simulink model "detection_and_isolation_v3"  (R2018a)
settings: Solver=ode45  StartTime=0.0  StopTime=0.8  RelTol=1e-3
values from neighbouring files (symbols this model uses):
  Ad = sysd.A    [SimulinkInit.m]
  Bd = sysd.B    [SimulinkInit.m]
  C1 = Cd(1,:)    [SimulinkInit.m]
  C2 = Cd(2,:)    [SimulinkInit.m]
  C3 = Cd(3,:)    [SimulinkInit.m]
  C4 = Cd(4,:)    [SimulinkInit.m]
  Cd = sysd.C    [SimulinkInit.m]
  T1 = 0.4    [parametros_BIO.m]
  T2 = 1    [parametros_BIO.m]
  T3 = 15    [parametros_BIO.m]
  T4 = 2.5    [parametros_BIO.m]
  T5 = 3.3    [parametros_BIO.m]
  tm = 1e-4    (= 0.0001)    [SimulinkInit.m]
undefined symbols (not defined in the file or in its folder): C10, C11, C12, C5, C6, C7, C8, C9, F1, F10, F11, F12, F2, F3, F4, F5, F6, F7, F8, F9, H1, H10, H11, H12, H2, H3, H4, H5, H6, H7, H8, H9, K10U, K11U, K12U, K1U, K2U, K3U, K4U, K5U, K6U, K7U, K8U, K9U, T10, T11, T12, T6, T7, T8, T9
libraries: dsparch4 x2, powerlib_meascontrol x2, dspstat3 x2, dspmlti4 x1
settings Model: Creator=cmparedes  LastModifiedBy=cmparedes

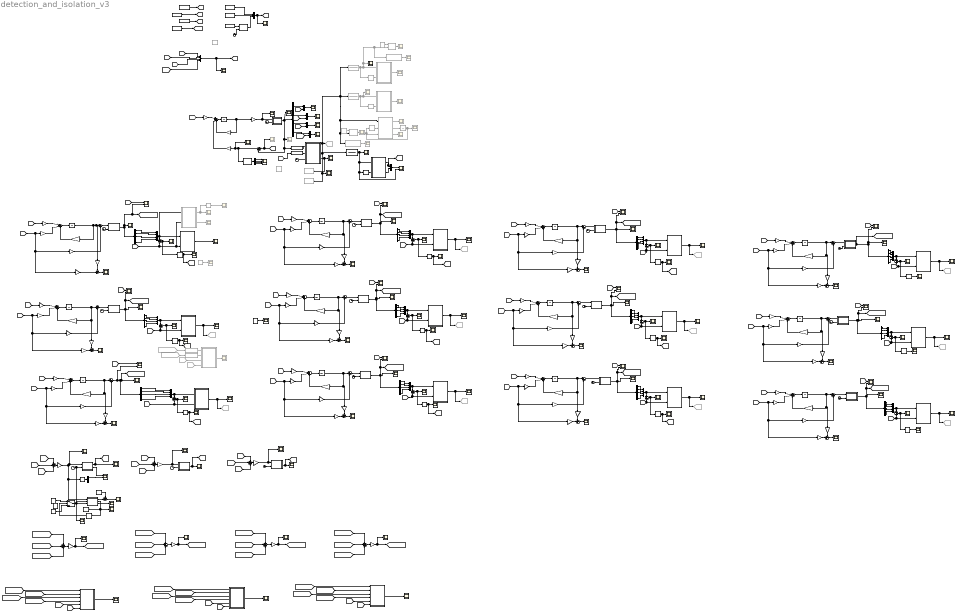
== system detection_and_isolation_v3 ==
  Abs : Abs
  Array From Workspace1 : FromWorkspace  VariableName=[tiempo,I2]  SampleTime=tm
  Array From Workspace2 : FromWorkspace  VariableName=[tiempo,I1]  SampleTime=tm
  Array From Workspace3 : FromWorkspace  VariableName=[tiempo,I3]  SampleTime=tm
  Array From Workspace4 : FromWorkspace  VariableName=[tiempo,V_load]  SampleTime=tm
  Array From Workspace5 : FromWorkspace  VariableName=[tiempo,u1]  SampleTime=tm
  Array From Workspace6 : FromWorkspace  VariableName=[tiempo,u2]  SampleTime=tm
  Array From Workspace7 : FromWorkspace  VariableName=[tiempo,u3]  SampleTime=tm
  Clock{,1..16} (17 alike) : Clock
  Constant : Constant  Value=0
  Constant1 : Constant
  Constant2 : Constant
  Constant3 : Constant
  Constant8 : Constant  Commented=on  Value=10
  Constant9 : Constant  Commented=on  Value=10
  DWT : dspmlti4/Dyadic Analysis Filter Bank  Commented=on  Wname=User-defined  OrdRec_ordDec=[1 / 1]  Order=2  LPF="[0.0352   -0.0854   -0.1350   0.4599   0.8069   0.3327]"  HPF="[-0.3327    0.8069   -0.4599   -0.1350    0.0854    0.0352]"  NumLevels=2  tree=Symmetric  Output=Single port  OutputFrames=off
      settings: SourceProductName=DSP System Toolbox  SourceProductBaseCode=DS
  Delay : Delay  Commented=on  DelayLength=1
  Delay1 : Delay  Commented=on  DelayLength=1
  Delay2 : Delay  DelayLength=1
  Delay3 : Delay  Commented=on  DelayLength=1
  Delay4 : Delay  DelayLength=1
  Demux : Demux
  Demux{1,3..13} (12 alike) : Demux  Outputs=5
  Demux19 : Demux
  Demux2 : Demux
  Derivative{,1..2,4..12} (12 alike) : Derivative  CoefficientInTFapproximation=0
  Derivative13 : Derivative  Commented=on  CoefficientInTFapproximation=0
  Derivative3 : Derivative
  From54 : From  Commented=on  GotoTag=x_hat_uio1
  From55 : From  Commented=on  GotoTag=x_hat_uio2
  From56 : From  Commented=on  GotoTag=rol
  From57 : From  Commented=on  GotoTag=ruo2
  Gain{,1..6} (7 alike) : Gain  Gain=1/3
  Goto{5,7,9,11,13,15,17,19,36} (9 alike) : Goto  Commented=on  GotoTag=ruo4
  Goto28 : Goto  Commented=on  GotoTag=ruo2
  Goto31 : Goto  Commented=on  GotoTag=ruo3
  Goto35 : Goto  Commented=on  GotoTag=rol
  Hw4 : dsparch4/Analog Filter Design  Commented=on  method=Bessel  filttype=Lowpass  N=2  Wlo=7000*2*pi  Whi=80  Rp=2  Rs=80
  Hw5 : dsparch4/Analog Filter Design  Commented=on  method=Bessel  filttype=Lowpass  N=20  Wlo=60*2*pi  Whi=80  Rp=2  Rs=80
  Integrator : Integrator  Commented=on
  MATLAB Function : MATLAB Function  TreatAsAtomicUnit=on
  MATLAB Function1 : MATLAB Function  TreatAsAtomicUnit=on
  MATLAB Function10 : MATLAB Function  TreatAsAtomicUnit=on
  MATLAB Function11 : MATLAB Function  Commented=on  TreatAsAtomicUnit=on
  MATLAB Function12 : MATLAB Function  TreatAsAtomicUnit=on
  MATLAB Function13 : MATLAB Function  TreatAsAtomicUnit=on
  MATLAB Function14 : MATLAB Function  Commented=on  TreatAsAtomicUnit=on
  MATLAB Function15 : MATLAB Function  TreatAsAtomicUnit=on
  MATLAB Function16 : MATLAB Function  TreatAsAtomicUnit=on
  MATLAB Function17 : MATLAB Function  TreatAsAtomicUnit=on
  MATLAB Function18 : MATLAB Function  TreatAsAtomicUnit=on
  MATLAB Function19 : MATLAB Function  TreatAsAtomicUnit=on
  MATLAB Function2 : MATLAB Function  TreatAsAtomicUnit=on
  MATLAB Function20 : MATLAB Function  TreatAsAtomicUnit=on
  MATLAB Function21 : MATLAB Function  TreatAsAtomicUnit=on
  MATLAB Function22 : MATLAB Function  TreatAsAtomicUnit=on
  MATLAB Function23 : MATLAB Function  TreatAsAtomicUnit=on
  MATLAB Function24 : MATLAB Function  TreatAsAtomicUnit=on
  MATLAB Function25 : MATLAB Function  TreatAsAtomicUnit=on
  MATLAB Function26 : MATLAB Function  TreatAsAtomicUnit=on
  MATLAB Function27 : MATLAB Function  TreatAsAtomicUnit=on
  MATLAB Function28 : MATLAB Function  TreatAsAtomicUnit=on
  MATLAB Function29 : MATLAB Function  TreatAsAtomicUnit=on
  MATLAB Function3 : MATLAB Function  TreatAsAtomicUnit=on
  MATLAB Function30 : MATLAB Function  TreatAsAtomicUnit=on
  MATLAB Function31 : MATLAB Function  TreatAsAtomicUnit=on
  MATLAB Function32 : MATLAB Function  TreatAsAtomicUnit=on
  MATLAB Function33 : MATLAB Function  TreatAsAtomicUnit=on
  MATLAB Function34 : MATLAB Function  TreatAsAtomicUnit=on
  MATLAB Function35 : MATLAB Function  TreatAsAtomicUnit=on
  MATLAB Function36 : MATLAB Function  TreatAsAtomicUnit=on
  MATLAB Function37 : MATLAB Function  TreatAsAtomicUnit=on
  MATLAB Function38 : MATLAB Function  TreatAsAtomicUnit=on
  MATLAB Function39 : MATLAB Function  TreatAsAtomicUnit=on
  MATLAB Function4 : MATLAB Function  Commented=on  TreatAsAtomicUnit=on
  MATLAB Function5 : MATLAB Function  Commented=on  TreatAsAtomicUnit=on
  MATLAB Function6 : MATLAB Function  Commented=on  TreatAsAtomicUnit=on
  MATLAB Function7 : MATLAB Function  TreatAsAtomicUnit=on
  MATLAB Function8 : MATLAB Function  TreatAsAtomicUnit=on
  MATLAB Function9 : MATLAB Function  TreatAsAtomicUnit=on
  Mean (Variable Frequency) : powerlib_meascontrol/Measurements/Mean (Variable Frequency)  Commented=on  Finit=60  Fmin=45  Vinit=0  Ts=0
      settings: SourceProductName=Simscape Power Systems  SourceProductBaseCode=PS
  Mean (Variable Frequency)1 : powerlib_meascontrol/Measurements/Mean (Variable Frequency)  Commented=on  Finit=60  Fmin=45  Vinit=0  Ts=0
      settings: SourceProductName=Simscape Power Systems  SourceProductBaseCode=PS
  Median Filter : dspstat3/Median Filter  Commented=on  WindowLength=100  SimulateUsing=Interpreted execution
      settings: SourceProductName=DSP System Toolbox  SourceProductBaseCode=DS
  Median Filter1 : dspstat3/Median Filter  Commented=on  WindowLength=100  SimulateUsing=Interpreted execution
      settings: SourceProductName=DSP System Toolbox  SourceProductBaseCode=DS
  Memory : Memory
  Mux{1..6,8,13,15..19} (13 alike) : Mux
  Mux{9..12,14} (5 alike) : Mux  Inputs=2
  Mux7 : Mux  Inputs=3
  Scope{,1,4..7,9..13,15,23..25,27..32,34..39,41,44..56,58..77,84,93..104,106..122} (91 alike) : Scope
  Scope{2..3,8,14,16..22,26,33,40,57,92,105} (17 alike) : Scope  Commented=on
  Scope{42,78..83,85..91} (14 alike) : Scope  NumInputPorts=2
  Scope43 : Scope  NumInputPorts=4
  Signal Specification : SignalSpecification  Dimensions=4
  Signal Specification1 : SignalSpecification  Dimensions=4
  Signal Specification2 : SignalSpecification  Commented=on  Dimensions=3
  Signal Specification3 : SignalSpecification  Commented=on  Dimensions=3
  Sum{,3,7,15,18,22,30,34,36,42,46,48} (12 alike) : Sum  Inputs=|++
  Sum{1..2,5,11,13,20,26,28,32,38,40,44} (12 alike) : Sum  Inputs=+-
  Sum10 : Sum  Inputs=|+-
  Sum{6,12,17,21,23..24,27,29,33,39,41,45} (12 alike) : Sum  Inputs=-+|
  Sum{4,8..9,14,16,19,25,31,35,37,43,47,49} (13 alike) : Sum  Inputs=|+++  SampleTime=tm
  Sum{50..52,54..57} (7 alike) : Sum  Inputs=+++
  Sum53 : Sum  Inputs=+-|
  Switch : Switch  Criteria=u2 > Threshold
  To Workspace : ToWorkspace  Commented=on  VariableName=det  SampleTime=1e-4
  To Workspace1 : ToWorkspace  Commented=on  VariableName=norm  SampleTime=1e-4
  Transfer Fcn : TransferFcn  Commented=on  Denominator=[0.025 1]
  Transfer Fcn5 : TransferFcn  Commented=on  Denominator=[0.0025 1]
  Transfer Fcn6 : TransferFcn  Denominator=[0.005 1]
  Unit Delay{1..13} (13 alike) : UnitDelay  SampleTime=tm
  adis1 : Gain  Gain=F3  Multiplication=Matrix(K*u) (u vector)  SampleTime=tm
  adis10 : Gain  Gain=Ld'  Multiplication=Matrix(K*u) (u vector)  SampleTime=tm
  adis11 : Gain  Gain=F1  Multiplication=Matrix(K*u) (u vector)  SampleTime=tm
  adis12 : Gain  Gain=F2  Multiplication=Matrix(K*u) (u vector)  SampleTime=tm
  adis13 : Gain  Gain=F11  Multiplication=Matrix(K*u) (u vector)  SampleTime=tm
  adis14 : Gain  Gain=F12  Multiplication=Matrix(K*u) (u vector)  SampleTime=tm
  adis2 : Gain  Gain=F4  Multiplication=Matrix(K*u) (u vector)  SampleTime=tm
  adis3 : Gain  Gain=F5  Multiplication=Matrix(K*u) (u vector)  SampleTime=tm
  adis4 : Gain  Gain=F6  Multiplication=Matrix(K*u) (u vector)  SampleTime=tm
  adis5 : Gain  Gain=F7  Multiplication=Matrix(K*u) (u vector)  SampleTime=tm
  adis6 : Gain  Gain=F8  Multiplication=Matrix(K*u) (u vector)  SampleTime=tm
  adis7 : Gain  Gain=Ad  Multiplication=Matrix(K*u) (u vector)  SampleTime=tm
  adis8 : Gain  Gain=F9  Multiplication=Matrix(K*u) (u vector)  SampleTime=tm
  adis9 : Gain  Gain=F10  Multiplication=Matrix(K*u) (u vector)  SampleTime=tm
  bdis1 : Gain  Gain=T3*Bd  Multiplication=Matrix(K*u) (u vector)  SampleTime=tm
  bdis10 : Gain  Gain=T2*Bd  Multiplication=Matrix(K*u) (u vector)  SampleTime=tm
  bdis11 : Gain  Gain=K2U  Multiplication=Matrix(K*u) (u vector)  SampleTime=tm
  bdis12 : Gain  Gain=H2  Multiplication=Matrix(K*u) (u vector)  SampleTime=tm
  bdis13 : Gain  Gain=eye(1)-C2*H2  Multiplication=Matrix(K*u) (u vector)  SampleTime=tm
  bdis14 : Gain  Gain=eye(1)-C1*H1  Multiplication=Matrix(K*u) (u vector)  SampleTime=tm
  bdis15 : Gain  Gain=C1  Multiplication=Matrix(K*u) (u vector)  SampleTime=tm
  bdis16 : Gain  Gain=C2  Multiplication=Matrix(K*u) (u vector)  SampleTime=tm
  bdis17 : Gain  Gain=T4*Bd  Multiplication=Matrix(K*u) (u vector)  SampleTime=tm
  bdis18 : Gain  Gain=K4U  Multiplication=Matrix(K*u) (u vector)  SampleTime=tm
  bdis19 : Gain  Gain=H4  Multiplication=Matrix(K*u) (u vector)  SampleTime=tm
  bdis2 : Gain  Gain=K3U  Multiplication=Matrix(K*u) (u vector)  SampleTime=tm
  bdis20 : Gain  Gain=eye(1)-C4*H4  Multiplication=Matrix(K*u) (u vector)  SampleTime=tm
  bdis21 : Gain  Gain=C4  Multiplication=Matrix(K*u) (u vector)  SampleTime=tm
  bdis22 : Gain  Gain=T5*Bd  Multiplication=Matrix(K*u) (u vector)  SampleTime=tm
  bdis23 : Gain  Gain=K5U  Multiplication=Matrix(K*u) (u vector)  SampleTime=tm
  bdis24 : Gain  Gain=H5  Multiplication=Matrix(K*u) (u vector)  SampleTime=tm
  bdis25 : Gain  Gain=eye(1)-C5*H5  Multiplication=Matrix(K*u) (u vector)  SampleTime=tm
  bdis26 : Gain  Gain=C5  Multiplication=Matrix(K*u) (u vector)  SampleTime=tm
  bdis27 : Gain  Gain=T6*Bd  Multiplication=Matrix(K*u) (u vector)  SampleTime=tm
  bdis28 : Gain  Gain=K6U  Multiplication=Matrix(K*u) (u vector)  SampleTime=tm
  bdis29 : Gain  Gain=H6  Multiplication=Matrix(K*u) (u vector)  SampleTime=tm
  bdis3 : Gain  Gain=H3  Multiplication=Matrix(K*u) (u vector)  SampleTime=tm
  bdis30 : Gain  Gain=eye(1)-C6*H6  Multiplication=Matrix(K*u) (u vector)  SampleTime=tm
  bdis31 : Gain  Gain=C6  Multiplication=Matrix(K*u) (u vector)  SampleTime=tm
  bdis32 : Gain  Gain=T7*Bd  Multiplication=Matrix(K*u) (u vector)  SampleTime=tm
  bdis33 : Gain  Gain=K7U  Multiplication=Matrix(K*u) (u vector)  SampleTime=tm
  bdis34 : Gain  Gain=H7  Multiplication=Matrix(K*u) (u vector)  SampleTime=tm
  bdis35 : Gain  Gain=eye(1)-C7*H7  Multiplication=Matrix(K*u) (u vector)  SampleTime=tm
  bdis36 : Gain  Gain=C7  Multiplication=Matrix(K*u) (u vector)  SampleTime=tm
  bdis37 : Gain  Gain=T8*Bd  Multiplication=Matrix(K*u) (u vector)  SampleTime=tm
  bdis38 : Gain  Gain=K8U  Multiplication=Matrix(K*u) (u vector)  SampleTime=tm
  bdis39 : Gain  Gain=H8  Multiplication=Matrix(K*u) (u vector)  SampleTime=tm
  bdis4 : Gain  Gain=eye(1)-C3*H3  Multiplication=Matrix(K*u) (u vector)  SampleTime=tm
  bdis40 : Gain  Gain=eye(1)-C8*H8  Multiplication=Matrix(K*u) (u vector)  SampleTime=tm
  bdis41 : Gain  Gain=C8  Multiplication=Matrix(K*u) (u vector)  SampleTime=tm
  bdis42 : Gain  Gain=T9*Bd  Multiplication=Matrix(K*u) (u vector)  SampleTime=tm
  bdis43 : Gain  Gain=K9U  Multiplication=Matrix(K*u) (u vector)  SampleTime=tm
  bdis44 : Gain  Gain=H9  Multiplication=Matrix(K*u) (u vector)  SampleTime=tm
  bdis45 : Gain  Gain=eye(1)-C9*H9  Multiplication=Matrix(K*u) (u vector)  SampleTime=tm
  bdis46 : Gain  Gain=C9  Multiplication=Matrix(K*u) (u vector)  SampleTime=tm
  bdis47 : Gain  Gain=T10*Bd  Multiplication=Matrix(K*u) (u vector)  SampleTime=tm
  bdis48 : Gain  Gain=K10U  Multiplication=Matrix(K*u) (u vector)  SampleTime=tm
  bdis49 : Gain  Gain=H10  Multiplication=Matrix(K*u) (u vector)  SampleTime=tm
  bdis5 : Gain  Gain=Bd  Multiplication=Matrix(K*u) (u vector)  SampleTime=tm
  bdis50 : Gain  Gain=eye(1)-C10*H10  Multiplication=Matrix(K*u) (u vector)  SampleTime=tm
  bdis51 : Gain  Gain=C10  Multiplication=Matrix(K*u) (u vector)  SampleTime=tm
  bdis52 : Gain  Gain=T11*Bd  Multiplication=Matrix(K*u) (u vector)  SampleTime=tm
  bdis53 : Gain  Gain=K11U  Multiplication=Matrix(K*u) (u vector)  SampleTime=tm
  bdis54 : Gain  Gain=H11  Multiplication=Matrix(K*u) (u vector)  SampleTime=tm
  bdis55 : Gain  Gain=eye(1)-C11*H11  Multiplication=Matrix(K*u) (u vector)  SampleTime=tm
  bdis56 : Gain  Gain=C11  Multiplication=Matrix(K*u) (u vector)  SampleTime=tm
  bdis57 : Gain  Gain=T12*Bd  Multiplication=Matrix(K*u) (u vector)  SampleTime=tm
  bdis58 : Gain  Gain=K12U  Multiplication=Matrix(K*u) (u vector)  SampleTime=tm
  bdis59 : Gain  Gain=H12  Multiplication=Matrix(K*u) (u vector)  SampleTime=tm
  bdis6 : Gain  Gain=C3  Multiplication=Matrix(K*u) (u vector)  SampleTime=tm
  bdis60 : Gain  Gain=eye(1)-C12*H12  Multiplication=Matrix(K*u) (u vector)  SampleTime=tm
  bdis61 : Gain  Gain=C12  Multiplication=Matrix(K*u) (u vector)  SampleTime=tm
  bdis7 : Gain  Gain=T1*Bd  Multiplication=Matrix(K*u) (u vector)  SampleTime=tm
  bdis8 : Gain  Gain=K1U  Multiplication=Matrix(K*u) (u vector)  SampleTime=tm
  bdis9 : Gain  Gain=H1  Multiplication=Matrix(K*u) (u vector)  SampleTime=tm
  cdis4 : Gain  Gain=Cd  Multiplication=Matrix(K*u) (u vector)  SampleTime=tm
  wires:
  adis7/1 -> Sum8/3
  Demux19/1 -> Scope43/1
  [u_fs] -> bdis5/1
  Signal Specification/1 -> MATLAB Function3/1(y_hat)
  [y_ma] -> Scope33/1, Sum10/1
  bdis5/1 -> Sum8/1
  [I3] -> Mux11/2
  Demux2/3 -> Mux11/1
  Mux9/1 -> Scope31/1
  Demux2/2 -> Mux10/1
  MATLAB Function7/2(Th_det) -> Mux14/2
  From56/1 -> MATLAB Function11/4(rol)
  adis11/1 -> Sum14/3
  bdis11/1 -> Sum16/2
  Mux10/1 -> Scope32/1
  Sum14/1 -> Unit Delay7/1
  bdis12/1 -> Sum15/2
  MATLAB Function4/1(rol) -> Scope8/1
  [u_fs] -> bdis10/1
  Mux12/1 -> Scope34/1
  [I3] -> bdis13/1, bdis12/1, bdis11/1
  MATLAB Function7/1(rol) -> [rol], Mux14/1
  Delay3/1 -> MATLAB Function5/2(x1)
  Unit Delay10/1 -> bdis16/1, adis12/1, Sum15/1
  Constant9/1 -> Mean (Variable Frequency)/1
  [I2] -> Mux10/2
  Median Filter/1 -> Scope17/1
  Transfer Fcn/1 -> Delay/1, MATLAB Function4/1(r), Scope14/1
  Sum10/1 -> MATLAB Function2/1(r), Scope37/1, adis10/1
  Clock/1 -> MATLAB Function1/2(t)
  MATLAB Function2/1(y) -> Demux19/1
  bdis15/1 -> Sum23/1
  Demux5/1 -> Mux16/1
  Unit Delay2/1 -> bdis21/1, adis2/1, Sum7/1
  MATLAB Function5/1(rol) -> Scope21/1
  MATLAB Function8/1(ruo1) -> Scope54/1
  From55/1 -> Signal Specification3/1
  MATLAB Function5/2(xp) -> Integrator/1
  Delay/1 -> MATLAB Function4/2(r1)
  adis1/1 -> Sum4/3
  [y_ma] -> Signal Specification1/1
  bdis18/1 -> Sum9/2
  Mux7/1 -> Scope84/1, [u_fs]
  bdis17/1 -> Sum9/1
  Transfer Fcn6/1 -> Scope42/2, Delay2/1, MATLAB Function7/1(r), Scope41/1
  Demux19/2 -> Scope43/2
  MATLAB Function11/1(v2) -> Scope57/1
  From57/1 -> MATLAB Function11/3(ruo2)
  Sum16/1 -> Unit Delay10/1
  Demux19/3 -> Scope43/3
  [I1] -> bdis20/1, bdis19/1, bdis18/1
  Mux18/1 -> Sum11/1, MATLAB Function13/1(ya)
  MATLAB Function5/3(m) -> Scope26/1
  Unit Delay7/1 -> adis11/1, bdis15/1, Sum/1
  Mux14/1 -> Scope42/1
  [u_fs] -> bdis7/1
  adis2/1 -> Sum9/3
  bdis7/1 -> Sum14/1
  Demux5/3 -> Mux16/3
  Demux7/2 -> Mux18/2
  Delay1/1 -> MATLAB Function6/2(r1)
  Sum9/1 -> Unit Delay2/1
  Sum12/1 -> Scope61/1
  Demux7/1 -> Mux18/1
  Unit Delay6/1 -> cdis4/1, adis7/1
  bdis21/1 -> Sum12/1
  bdis19/1 -> Sum7/2
  Sum4/1 -> Unit Delay1/1
  Signal Specification3/1 -> MATLAB Function11/2(x_hat2)
  bdis9/1 -> Sum/2
  Sum2/1 -> Derivative1/1, Scope46/1
  Demux7/5 -> Mux18/4
  Demux4/3 -> Mux15/3
  Demux4/1 -> Mux15/1
  [u_fs] -> bdis17/1
  MATLAB Function13/1(ruo4) -> Goto36/1, Scope60/1
  Sum11/1 -> Derivative4/1, Scope59/1
  bdis4/1 -> Sum6/2
  Mean (Variable Frequency)/1 -> Scope19/1
  [I2] -> bdis14/1, bdis9/1, bdis8/1
  Signal Specification1/1 -> MATLAB Function3/2(y_m)
  bdis2/1 -> Sum4/2
  Unit Delay1/1 -> bdis6/1, adis1/1, Sum3/1
  [y_ma] -> Sum11/2, MATLAB Function13/2(ym)
  bdis14/1 -> Sum23/2
  MATLAB Function12/1(ruo3) -> Goto31/1, Scope51/1
  Mux17/1 -> Sum5/1, MATLAB Function12/1(ya)
  bdis1/1 -> Sum4/1
  Constant8/1 -> Mean (Variable Frequency)1/1
  Sum3/1 -> Demux6/1, [x_hat_uio13], Scope49/1, Scope80/2
  [V_vsi] -> bdis4/1, bdis3/1, bdis2/1
  Mux15/1 -> MATLAB Function14/1(ya), Sum1/1, MATLAB Function8/1(ya)
  Clock1/1 -> MATLAB Function3/3(tiempo)
  [u_fs] -> bdis1/1
  Demux5/5 -> Mux16/4
  bdis8/1 -> Sum14/2
  Sum8/1 -> Unit Delay6/1
  Integrator/1 -> Delay3/1, MATLAB Function5/3(x), Scope22/1
  Demux5/2 -> Mux16/2
  Demux6/5 -> Mux17/4
  bdis20/1 -> Sum12/2
  Mux11/1 -> Scope38/1
  Demux6/2 -> Mux17/2
  bdis6/1 -> Sum6/1
  bdis3/1 -> Sum3/2
  [y_ma] -> Sum5/2, MATLAB Function12/2(ym)
  adis12/1 -> Sum16/3
  [y_ma] -> Sum2/2, MATLAB Function9/2(ym)
  Mux16/1 -> Sum2/1, MATLAB Function9/1(ya)
  Demux4/5 -> Mux15/4
  [y_ma] -> Sum1/2, MATLAB Function14/2(ym), MATLAB Function8/2(ym)
  Demux6/3 -> Mux17/3
  bdis13/1 -> Sum24/2
  Sum6/1 -> Scope55/1
  Delay2/1 -> MATLAB Function7/2(r1)
  bdis10/1 -> Sum16/1
  MATLAB Function9/1(ruo2) -> Goto28/1, Scope48/1
  Demux2/1 -> Mux9/1
  Mean (Variable Frequency)1/1 -> Scope20/1
  Demux2/4 -> Mux12/1
  From54/1 -> Signal Specification2/1
  Sum24/1 -> Scope53/1
  Median Filter1/1 -> Scope18/1
  bdis16/1 -> Sum24/1
  MATLAB Function6/1(rol) -> Scope16/1
  Sum5/1 -> Derivative2/1, Scope50/1
  Sum23/1 -> Scope52/1
  [I1] -> Mux9/2
  [V_vsi] -> Mux12/2
  Transfer Fcn5/1 -> Delay1/1, MATLAB Function6/1(r), Median Filter1/1, Mean (Variable Frequency)1/2, Scope15/1
  Demux4/2 -> Mux15/2
  MATLAB Function1/1(y) -> Scope1/1, Demux2/1, Scope40/1, Sum10/2, Signal Specification/1
  MATLAB Function3/2(norm_rd) -> To Workspace1/1, Scope39/1
  Demux6/1 -> Mux17/1
  cdis4/1 -> MATLAB Function1/1(y_hat), Scope35/1
  Demux7/3 -> Mux18/3
  Demux19/4 -> Scope43/4
  Signal Specification2/1 -> MATLAB Function11/1(x_hat1)
  MATLAB Function3/1(rol) -> MATLAB Function5/1(r), Median Filter/1, Mean (Variable Frequency)/2, Transfer Fcn5/1, Transfer Fcn/1, Goto35/1, To Workspace/1, Scope36/1, Transfer Fcn6/1
  adis10/1 -> Sum8/2
  Array From Workspace2/1 -> [I1]
  Array From Workspace1/1 -> [I2]
  Array From Workspace3/1 -> [I3]
  Array From Workspace4/1 -> [V_vsi]
  Array From Workspace6/1 -> Mux7/2
  Array From Workspace5/1 -> Mux7/1
  MATLAB Function14/1(r) -> Derivative13/1, Scope2/1
  MATLAB Function14/2(r2) -> Scope3/1
  [u_fs] -> bdis22/1
  adis3/1 -> Sum19/3
  MATLAB Function15/1(ruo4) -> Goto5/1, Scope6/1
  Sum13/1 -> Derivative5/1, Scope5/1
  Mux1/1 -> Sum13/1, MATLAB Function15/1(ya)
  Sum17/1 -> Scope7/1
  Unit Delay3/1 -> bdis26/1, adis3/1, Sum18/1
  [I3] -> bdis25/1, bdis24/1, bdis23/1
  bdis26/1 -> Sum17/1
  bdis24/1 -> Sum18/2
  [y_ma] -> Sum13/2, MATLAB Function15/2(ym)
  Sum19/1 -> Unit Delay3/1
  bdis23/1 -> Sum19/2
  Demux1/5 -> Mux1/4
  Demux1/2 -> Mux1/2
  Demux1/3 -> Mux1/3
  Demux1/1 -> Mux1/1
  bdis25/1 -> Sum17/2
  bdis22/1 -> Sum19/1
  [u_fs] -> bdis27/1
  adis4/1 -> Sum25/3
  MATLAB Function16/1(ruo4) -> Goto7/1, Scope11/1
  Sum20/1 -> Derivative6/1, Scope10/1
  Mux2/1 -> Sum20/1, MATLAB Function16/1(ya)
  Sum21/1 -> Scope12/1
  Unit Delay4/1 -> bdis31/1, adis4/1, Sum22/1
  [V_vsi] -> bdis30/1, bdis29/1, bdis28/1
  bdis31/1 -> Sum21/1
  bdis29/1 -> Sum22/2
  [y_ma] -> Sum20/2, MATLAB Function16/2(ym)
  Sum25/1 -> Unit Delay4/1
  bdis28/1 -> Sum25/2
  Demux3/5 -> Mux2/4
  Demux3/2 -> Mux2/2
  Demux3/3 -> Mux2/3
  Demux3/1 -> Mux2/1
  bdis30/1 -> Sum21/2
  bdis27/1 -> Sum25/1
  MATLAB Function18/1(ruo4) -> Goto11/1, Scope30/1
  Unit Delay8/1 -> bdis41/1, adis6/1, Sum30/1
  Mux3/1 -> Sum28/1, MATLAB Function18/1(ya)
  bdis44/1 -> Sum34/2
  bdis46/1 -> Sum33/1
  [V_vsi] -> bdis45/1, bdis44/1, bdis43/1
  Mux5/1 -> Sum32/1, MATLAB Function19/1(ya)
  Sum33/1 -> Scope24/1
  Sum32/1 -> Derivative9/1, Scope13/1
  MATLAB Function19/1(ruo4) -> Goto13/1, Scope23/1
  [u_fs] -> bdis42/1
  bdis45/1 -> Sum33/2
  bdis37/1 -> Sum31/1
  Demux9/3 -> Mux5/3
  bdis43/1 -> Sum35/2
  adis8/1 -> Sum35/3
  [u_fs] -> bdis32/1
  adis5/1 -> Sum37/3
  [y_ma] -> Sum32/2, MATLAB Function19/2(ym)
  Sum26/1 -> Derivative7/1, Scope29/1
  Sum27/1 -> Scope63/1
  Unit Delay5/1 -> bdis36/1, adis5/1, Sum36/1
  Unit Delay9/1 -> bdis46/1, adis8/1, Sum34/1
  [I1] -> bdis35/1, bdis34/1, bdis33/1
  bdis34/1 -> Sum36/2
  Sum28/1 -> Derivative8/1, Scope27/1
  Sum37/1 -> Unit Delay5/1
  bdis33/1 -> Sum37/2
  bdis40/1 -> Sum29/2
  bdis32/1 -> Sum37/1
  [I2] -> bdis40/1, bdis39/1, bdis38/1
  Sum29/1 -> Scope64/1
  Demux8/5 -> Mux3/4
  bdis38/1 -> Sum31/2
  Sum31/1 -> Unit Delay8/1
  Mux4/1 -> Sum26/1, MATLAB Function17/1(ya)
  [y_ma] -> Sum28/2, MATLAB Function18/2(ym)
  Demux10/5 -> Mux4/4
  bdis39/1 -> Sum30/2
  bdis41/1 -> Sum29/1
  Demux8/3 -> Mux3/3
  Demux8/2 -> Mux3/2
  bdis36/1 -> Sum27/1
  adis6/1 -> Sum31/3
  [u_fs] -> bdis37/1
  bdis35/1 -> Sum27/2
  Demux10/1 -> Mux4/1
  Demux9/5 -> Mux5/4
  MATLAB Function17/1(ruo4) -> Goto9/1, Scope62/1
  bdis42/1 -> Sum35/1
  Demux9/2 -> Mux5/2
  Sum35/1 -> Unit Delay9/1
  Demux10/2 -> Mux4/2
  Demux9/1 -> Mux5/1
  Demux10/3 -> Mux4/3
  Demux8/1 -> Mux3/1
  [y_ma] -> Sum26/2, MATLAB Function17/2(ym)
  MATLAB Function21/1(ruo4) -> Goto17/1, Scope73/1
  Unit Delay12/1 -> bdis56/1, adis13/1, Sum42/1
  Mux6/1 -> Sum40/1, MATLAB Function21/1(ya)
  bdis59/1 -> Sum46/2
  bdis61/1 -> Sum45/1
  [I3] -> bdis60/1, bdis59/1, bdis58/1
  Mux19/1 -> Sum44/1, MATLAB Function22/1(ya)
  Sum45/1 -> Scope68/1
  Sum44/1 -> Derivative12/1, Scope66/1
  MATLAB Function22/1(ruo4) -> Goto19/1, Scope67/1
  [u_fs] -> bdis57/1
  bdis60/1 -> Sum45/2
  bdis52/1 -> Sum43/1
  Demux12/3 -> Mux19/3
  bdis58/1 -> Sum47/2
  adis14/1 -> Sum47/3
  [u_fs] -> bdis47/1
  adis9/1 -> Sum49/3
  [y_ma] -> Sum44/2, MATLAB Function22/2(ym)
  Sum38/1 -> Derivative10/1, Scope72/1
  Sum39/1 -> Scope75/1
  Unit Delay11/1 -> bdis51/1, adis9/1, Sum48/1
  Unit Delay13/1 -> bdis61/1, adis14/1, Sum46/1
  [I1] -> bdis50/1, bdis49/1, bdis48/1
  bdis49/1 -> Sum48/2
  Sum40/1 -> Derivative11/1, Scope70/1
  Sum49/1 -> Unit Delay11/1
  bdis48/1 -> Sum49/2
  bdis55/1 -> Sum41/2
  bdis47/1 -> Sum49/1
  [I2] -> bdis55/1, bdis54/1, bdis53/1
  Sum41/1 -> Scope76/1
  Demux11/5 -> Mux6/4
  bdis53/1 -> Sum43/2
  Sum43/1 -> Unit Delay12/1
  Mux13/1 -> Sum38/1, MATLAB Function20/1(ya)
  [y_ma] -> Sum40/2, MATLAB Function21/2(ym)
  Demux13/5 -> Mux13/4
  bdis54/1 -> Sum42/2
  bdis56/1 -> Sum41/1
  Demux11/3 -> Mux6/3
  Demux11/2 -> Mux6/2
  bdis51/1 -> Sum39/1
  adis13/1 -> Sum43/3
  [u_fs] -> bdis52/1
  bdis50/1 -> Sum39/2
  Demux13/1 -> Mux13/1
  Demux12/5 -> Mux19/4
  MATLAB Function20/1(ruo4) -> Goto15/1, Scope74/1
  bdis57/1 -> Sum47/1
  Demux12/2 -> Mux19/2
  Sum47/1 -> Unit Delay13/1
  Demux13/2 -> Mux13/2
  Demux12/1 -> Mux19/1
  Demux13/3 -> Mux13/3
  Demux11/1 -> Mux6/1
  [y_ma] -> Sum38/2, MATLAB Function20/2(ym)
  Sum/1 -> MATLAB Function/1(u)
  [y_ma] -> Scope79/1
  [y_ma] -> Scope80/1
  [y_ma] -> Scope81/1
  [y_ma] -> Scope82/1
  [y_ma] -> Scope83/1
  Clock2/1 -> MATLAB Function23/2(t)
  Array From Workspace7/1 -> MATLAB Function23/1(y_hat)
  MATLAB Function23/1(y) -> Mux7/3
  [y_ma] -> Scope85/1
  [y_ma] -> Scope86/1
  [y_ma] -> Scope87/1
  [y_ma] -> Scope88/1
  [y_ma] -> Scope89/1
  [y_ma] -> Scope90/1
  [y_ma] -> Scope78/1
  MATLAB Function/1(y) -> Scope47/1, Scope78/2, [x_hat_uio11], Demux4/1
  Clock3/1 -> MATLAB Function/2(t)
  Clock4/1 -> MATLAB Function24/2(t)
  Sum15/1 -> MATLAB Function24/1(u)
  MATLAB Function24/1(y) -> Demux5/1, [x_hat_uio12], Scope79/2, Scope44/1
  Clock5/1 -> MATLAB Function25/2(t)
  Sum7/1 -> MATLAB Function25/1(u)
  MATLAB Function25/1(y) -> Scope58/1, [x_hat_uio21], Scope81/2, Demux7/1
  Clock6/1 -> MATLAB Function26/2(t)
  Sum18/1 -> MATLAB Function26/1(u)
  MATLAB Function26/1(y) -> Scope4/1, [x_hat_uio22], Scope82/2, Demux1/1
  Clock7/1 -> MATLAB Function27/2(t)
  Sum22/1 -> MATLAB Function27/1(u)
  MATLAB Function27/1(y) -> Demux3/1, [x_hat_uio23], Scope83/2, Scope9/1
  Clock8/1 -> MATLAB Function28/2(t)
  Sum36/1 -> MATLAB Function28/1(u)
  MATLAB Function28/1(y) -> Demux10/1, [x_hat_uio31], Scope85/2, Scope28/1
  Clock9/1 -> MATLAB Function29/2(t)
  Sum30/1 -> MATLAB Function29/1(u)
  MATLAB Function29/1(y) -> Demux8/1, [x_hat_uio32], Scope86/2, Scope25/1
  Clock10/1 -> MATLAB Function30/2(t)
  Sum34/1 -> MATLAB Function30/1(u)
  MATLAB Function30/1(y) -> Demux9/1, [x_hat_uio33], Scope87/2, Scope65/1
  Clock11/1 -> MATLAB Function31/2(t)
  Clock12/1 -> MATLAB Function32/2(t)
  Sum46/1 -> MATLAB Function32/1(u)
  MATLAB Function32/1(y) -> Demux12/1, [x_hat_uio43], Scope90/2, Scope77/1
  Sum48/1 -> MATLAB Function31/1(u)
  Clock13/1 -> MATLAB Function33/2(t)
  Sum42/1 -> MATLAB Function33/1(u)
  MATLAB Function33/1(y) -> Demux11/1, [x_hat_uio42], Scope89/2, Scope69/1
  Derivative1/1 -> [druo2], Scope93/1
  Derivative2/1 -> [druo3], Scope94/1
  Derivative3/1 -> Scope95/1
  Derivative4/1 -> [druo4], Scope96/1
  Derivative5/1 -> [druo5], Scope97/1
  Derivative6/1 -> [druo6], Scope98/1
  Derivative7/1 -> [druo7], Scope99/1
  Derivative8/1 -> [druo8], Scope100/1
  Derivative9/1 -> [druo9], Scope101/1
  Derivative10/1 -> Scope102/1
  Derivative11/1 -> Scope103/1
  Derivative12/1 -> Scope104/1
  Derivative/1 -> [druo1], Scope106/1
  Derivative13/1 -> Scope92/1
  Mux8/1 -> Scope/1, [y_ma]
  [I1] -> Mux8/1
  [I2] -> Mux8/2
  [I3] -> Mux8/3
  [V_vsi] -> Mux8/4
  Hw5/1 -> Scope105/1
  Sum1/1 -> Derivative/1, Scope45/1
  [druo2] -> Sum50/2
  [druo3] -> Sum50/3
  [druo1] -> Sum50/1
  Sum50/1 -> Gain/1
  Gain/1 -> MATLAB Function36/1(dr), Abs/1, MATLAB Function37/1(dr), Scope108/1
  [druo5] -> Sum51/2
  [druo4] -> Sum51/1
  Gain1/1 -> MATLAB Function34/1(dr), Scope110/1
  [druo6] -> Sum51/3
  Sum51/1 -> Gain1/1
  [druo8] -> Sum52/2
  [druo7] -> Sum52/1
  Gain2/1 -> MATLAB Function35/1(dr), Scope112/1
  [druo9] -> Sum52/3
  Sum52/1 -> Gain2/1
  Clock14/1 -> MATLAB Function37/2(t), MATLAB Function36/2(t)
  MATLAB Function37/1(r) -> [ruo1], Scope118/1
  MATLAB Function34/1(r) -> [ruo2], Scope107/1
  Clock15/1 -> MATLAB Function34/2(t)
  MATLAB Function35/1(r) -> [ruo3], Scope109/1
  Clock16/1 -> MATLAB Function35/2(t)
  MATLAB Function37/2(th) -> Scope91/1
  Constant1/1 -> Switch/3
  Constant/1 -> Switch/1
  Switch/1 -> Scope114/1, MATLAB Function36/3(ban)
  MATLAB Function36/2(c) -> Memory/1, Delay4/1, Scope113/1
  Abs/1 -> Demux/1
  Demux/1 -> Scope91/2
  MATLAB Function36/3(o) -> Scope115/1
  Sum53/1 -> Scope111/1
  MATLAB Function36/1(r) -> Sum53/2
  Constant3/1 -> Sum53/1
  Memory/1 -> Switch/2
  [ruo1] -> MATLAB Function38/5(ruo1)
  [rol] -> MATLAB Function38/6(rol)
  [x_hat_uio12] -> Sum54/2
  [x_hat_uio11] -> Sum54/1
  [x_hat_uio13] -> Sum54/3
  Sum54/1 -> Gain3/1
  Gain3/1 -> Scope56/1, [x_hat_uio1]
  [x_hat_uio1] -> MATLAB Function38/1(x_hat1)
  [x_hat_uio21] -> Sum55/1
  Gain4/1 -> Scope117/1, [x_hat_uio2]
  [x_hat_uio23] -> Sum55/3
  [x_hat_uio22] -> Sum55/2
  Sum55/1 -> Gain4/1
  [x_hat_uio2] -> MATLAB Function38/2(x_hat2)
  [x_hat_uio31] -> Sum56/1
  Gain5/1 -> Scope119/1, [x_hat_uio3]
  [x_hat_uio32] -> Sum56/2
  [x_hat_uio33] -> Sum56/3
  Sum56/1 -> Gain5/1
  [x_hat_uio41] -> Sum57/1
  Gain6/1 -> Scope120/1, [x_hat_uio4]
  [x_hat_uio42] -> Sum57/2
  [x_hat_uio43] -> Sum57/3
  Sum57/1 -> Gain6/1
  MATLAB Function31/1(y) -> [x_hat_uio41], Scope88/2, Scope71/1, Demux13/1
  [x_hat_uio3] -> MATLAB Function38/3(x_hat3)
  [x_hat_uio4] -> MATLAB Function38/4(x_hat4)
  MATLAB Function38/1(v1) -> Scope116/1
  [x_hat_uio2] -> MATLAB Function10/2(x_hat2)
  MATLAB Function10/1(v1) -> Scope121/1
  [ruo2] -> MATLAB Function10/5(ruo1)
  [x_hat_uio1] -> MATLAB Function10/1(x_hat1)
  [rol] -> MATLAB Function10/6(rol)
  [x_hat_uio3] -> MATLAB Function10/3(x_hat3)
  [x_hat_uio4] -> MATLAB Function10/4(x_hat4)
  [x_hat_uio2] -> MATLAB Function39/2(x_hat2)
  MATLAB Function39/1(v1) -> Scope122/1
  [ruo3] -> MATLAB Function39/5(ruo1)
  [x_hat_uio1] -> MATLAB Function39/1(x_hat1)
  [rol] -> MATLAB Function39/6(rol)
  [x_hat_uio3] -> MATLAB Function39/3(x_hat3)
  [x_hat_uio4] -> MATLAB Function39/4(x_hat4)

== matlab function detection_and_isolation_v3/MATLAB Function14 ==
  data: ya input; r output; ym input; r2 output
function [r,r2] = fcn(ya,ym)
% yol=[u1 ; u2];
% ym=[ym1 ; ym2];

% rd1=ya1-ym1;
% rd2=ya2-ym2;

% ya=[ya(1:3)y(5)];
rd=ya-ym;
r=mean(ya)-mean(ym);%-mean(ya-ym); %sqrt(sum(rd.^2));
r2=mean(ya(1))-mean(ym(1));
% r2=ym(1)-mean(ym(1));

% if abs(r(1))  >= Th_uio_on && abs(r(2))  <= Th_uio_off && abs(r(3))  <= Th_uio_off && abs(r(4))  <= Th_uio_off
%     ruo1=1;
% else
%     ruo1=0;
% end

== matlab function detection_and_isolation_v3/MATLAB Function15 ==
  data: ya input; ruo4 output; ym input
function ruo4 = fcn(ya,ym)
Th_uio_on = 3e-3;
Th_uio_off = 1e-5;


Th_uio_on = 6e-3;


% yol=[u1 ; u2];
% ym=[ym1 ; ym2];

% rd1=ya1-ym1;
% rd2=ya2-ym2;

% ya=[ya(1:3)y(5)];
r=ya-ym;

if abs(r(1))  >= Th_uio_on && abs(r(2))  <= Th_uio_off && abs(r(3))  <= Th_uio_off && abs(r(4))  <= Th_uio_off
    ruo4=1;
else
    ruo4=0;
end

== matlab function detection_and_isolation_v3/MATLAB Function16 ==
  data: ya input; ruo4 output; ym input
function ruo4 = fcn(ya,ym)
Th_uio_on = 3e-3;
Th_uio_off = 1e-5;


Th_uio_on = 6e-3;


% yol=[u1 ; u2];
% ym=[ym1 ; ym2];

% rd1=ya1-ym1;
% rd2=ya2-ym2;

% ya=[ya(1:3)y(5)];
r=ya-ym;

if abs(r(1))  >= Th_uio_on && abs(r(2))  <= Th_uio_off && abs(r(3))  <= Th_uio_off && abs(r(4))  <= Th_uio_off
    ruo4=1;
else
    ruo4=0;
end

== matlab function detection_and_isolation_v3/MATLAB Function17 ==
  data: ya input; ruo4 output; ym input
function ruo4 = fcn(ya,ym)
Th_uio_on = 3e-3;
Th_uio_off = 1e-5;


Th_uio_on = 6e-3;


% yol=[u1 ; u2];
% ym=[ym1 ; ym2];

% rd1=ya1-ym1;
% rd2=ya2-ym2;

% ya=[ya(1:3)y(5)];
r=ya-ym;

if abs(r(1))  >= Th_uio_on && abs(r(2))  <= Th_uio_off && abs(r(3))  <= Th_uio_off && abs(r(4))  <= Th_uio_off
    ruo4=1;
else
    ruo4=0;
end

== matlab function detection_and_isolation_v3/MATLAB Function18 ==
  data: ya input; ruo4 output; ym input
function ruo4 = fcn(ya,ym)
Th_uio_on = 3e-3;
Th_uio_off = 1e-5;


Th_uio_on = 6e-3;


% yol=[u1 ; u2];
% ym=[ym1 ; ym2];

% rd1=ya1-ym1;
% rd2=ya2-ym2;

% ya=[ya(1:3)y(5)];
r=ya-ym;

if abs(r(1))  >= Th_uio_on && abs(r(2))  <= Th_uio_off && abs(r(3))  <= Th_uio_off && abs(r(4))  <= Th_uio_off
    ruo4=1;
else
    ruo4=0;
end

== matlab function detection_and_isolation_v3/MATLAB Function19 ==
  data: ya input; ruo4 output; ym input
function ruo4 = fcn(ya,ym)
Th_uio_on = 3e-3;
Th_uio_off = 1e-5;


Th_uio_on = 6e-3;


% yol=[u1 ; u2];
% ym=[ym1 ; ym2];

% rd1=ya1-ym1;
% rd2=ya2-ym2;

% ya=[ya(1:3)y(5)];
r=ya-ym;

if abs(r(1))  >= Th_uio_on && abs(r(2))  <= Th_uio_off && abs(r(3))  <= Th_uio_off && abs(r(4))  <= Th_uio_off
    ruo4=1;
else
    ruo4=0;
end

== matlab function detection_and_isolation_v3/MATLAB Function20 ==
  data: ya input; ruo4 output; ym input
function ruo4 = fcn(ya,ym)
Th_uio_on = 3e-3;
Th_uio_off = 1e-5;


Th_uio_on = 6e-3;


% yol=[u1 ; u2];
% ym=[ym1 ; ym2];

% rd1=ya1-ym1;
% rd2=ya2-ym2;

% ya=[ya(1:3)y(5)];
r=ya-ym;

if abs(r(1))  >= Th_uio_on && abs(r(2))  <= Th_uio_off && abs(r(3))  <= Th_uio_off && abs(r(4))  <= Th_uio_off
    ruo4=1;
else
    ruo4=0;
end

== matlab function detection_and_isolation_v3/MATLAB Function21 ==
  data: ya input; ruo4 output; ym input
function ruo4 = fcn(ya,ym)
Th_uio_on = 3e-3;
Th_uio_off = 1e-5;


Th_uio_on = 6e-3;


% yol=[u1 ; u2];
% ym=[ym1 ; ym2];

% rd1=ya1-ym1;
% rd2=ya2-ym2;

% ya=[ya(1:3)y(5)];
r=ya-ym;

if abs(r(1))  >= Th_uio_on && abs(r(2))  <= Th_uio_off && abs(r(3))  <= Th_uio_off && abs(r(4))  <= Th_uio_off
    ruo4=1;
else
    ruo4=0;
end

== matlab function detection_and_isolation_v3/MATLAB Function22 ==
  data: ya input; ruo4 output; ym input
function ruo4 = fcn(ya,ym)
Th_uio_on = 3e-3;
Th_uio_off = 1e-5;


Th_uio_on = 6e-3;


% yol=[u1 ; u2];
% ym=[ym1 ; ym2];

% rd1=ya1-ym1;
% rd2=ya2-ym2;

% ya=[ya(1:3)y(5)];
r=ya-ym;

if abs(r(1))  >= Th_uio_on && abs(r(2))  <= Th_uio_off && abs(r(3))  <= Th_uio_off && abs(r(4))  <= Th_uio_off
    ruo4=1;
else
    ruo4=0;
end

== matlab function detection_and_isolation_v3/MATLAB Function23 ==
  data: y_hat input; y output; t input
function y = fcn(y_hat,t)%u1,u2,ym1,ym2)
% if y_hat(3)>0
%     y_hat(3)=y_hat(3)*1.38;
%     %     y_hat(3)=y_hat(3)+10;
% end


if t>=0.33*100
    y=y_hat+5;
else
    y=y_hat;
end

== matlab function detection_and_isolation_v3/MATLAB Function4 ==
  data: r input; rol output; r1 input
function rol = fcn(r,r1)%u1,u2,ym1,ym2)
Th_det = 6.5e-8;
Th_det=0.1;  %2.5

m=r-r1;
if m>0
    Th_det=0.1;  %2.5
elseif m<0 && r<=0.1
    Th_det=0.9; 
end


% sys=tf(1,[0.001 1]);


if r >=Th_det
    rol=1;
else
    rol=0;
end

== matlab function detection_and_isolation_v3/MATLAB Function3 ==
  data: y_hat input; rol output; y_m input; norm_rd output; tiempo input
function [rol,norm_rd] = fcn(y_hat,y_m,tiempo)%u1,u2,ym1,ym2)
Th_det = 6.5e-8;
Th_det=0.07;%2.3e-2; %Funciona bien si los pulsos no estan tan separados
Th_det_up=1;  %2.5 2.25
Th_det_down=-1;
if tiempo >=0.0015 && tiempo <=0.35
    Th_det_up=2.23e-2;  %2.5 2.25
    Th_det_down=3e-4;
else
    Th_det_up=2.25e-2;  %2.5 2.25
    Th_det_down=3e-3;
end
% Th_det=38;
% yol=[u1 ; u2];
% ym=[ym1 ; ym2];

rd1=(y_hat(1)-y_m(1))/100;%200;
rd2=(y_hat(2)-y_m(2))/120;%500;
rd3=(y_hat(3)-y_m(3))/400;%1300; 
rd4=(y_hat(4)-y_m(4))/500;

% rd=y_hat-y_m;
rd=[rd1 rd2 rd3 rd4];
norm_rd=sqrt(sum(rd.^2));
% sys=tf(1,[0.001 1]);


if norm_rd >=Th_det%Th_det_up && norm_rd <=Th_det_down
    rol=1;
else
    rol=0;
end

== matlab function detection_and_isolation_v3/MATLAB Function1 ==
  data: y_hat input; y output; t input
function y = fcn(y_hat,t)%u1,u2,ym1,ym2)
if y_hat(3)>0
    y_hat(3)=y_hat(3)*1.38;
    %     y_hat(3)=y_hat(3)+10;
end

% if t<=0.33
%     y1=y_hat(1)*1;%0.92;
%     y2=y_hat(2)*1;
%     y3=y_hat(3)*1;%1.1; 0.71 0.77 +28
% %     if y3<0
% %         y3=y3+11;
% %     end
%     y4=y_hat(4)*1;%y_hat(4)*1;
%
%
%
% else
%     y1=y_hat(1)*1;%0.92;
%     y2=y_hat(2)*1;
%     y3=y_hat(3)*0.4;%1.1; 0.65; 0.5
%     y4=y_hat(4)*1;%y_hat(4)*1;
% end
if t<=0.33
    y1=y_hat(1)*0.85;
    y2=y_hat(2)*0.8; %0.85
    y3=y_hat(3)*0.57; %0.6
    y4=y_hat(4)*0.88; %0.9
else
    y1=y_hat(1)*0.98;
    y2=y_hat(2)*1.16; %1.13  1.16
    y3=y_hat(3)*0.45; %0.5
    y4=y_hat(4);
    
end

y=[y1 y2 y3 y4];
% if norm_rd >=Th_det
%     rol=1;
% else
%     rol=0;
% end

== matlab function detection_and_isolation_v3/MATLAB Function2 ==
  data: r input; y output
function y = fcn(r)%u1,u2,ym1,ym2)

r1=r(1)/2000;%200;
r2=r(2)/2000;%500;
r3=r(3)/2000;%1300;
r4=r(4)/2000;
y=[r1 r2 r3 r4];
% if norm_rd >=Th_det
%     rol=1;
% else
%     rol=0;
% end

== matlab function detection_and_isolation_v3/MATLAB Function ==
  data: u input; y output; t input
function y = fcn(u,t)
y1=u(1);
y2=u(2);
if t<=0.33
    y3=u(3)*0.69;%*0.52;
else
    y3=u(3)*0.52;
end
y4=u(4);
y5=u(5);
y = [y1 y2 y3 y4 y5];

== matlab function detection_and_isolation_v3/MATLAB Function24 ==
  data: u input; y output; t input
function y = fcn(u,t)
y1=u(1);
y2=u(2);
if t>0.33
    y2=u(2)*1.31;%*0.52;
    y5=u(5)*1.55;
else
    y2=u(2);
    
    y5=u(5)*1.39;
    
end
y3=u(3);
y4=u(4);


y = [y1 y2 y3 y4 y5];

== matlab function detection_and_isolation_v3/MATLAB Function25 ==
  data: u input; y output; t input
function y = fcn(u,t)
y1=u(1);
y2=u(2);
if t>0.33
    y3=u(3)*0.54+5;
    y5=u(5)*1.15;
else
    y3=u(3)*0.7;
    
    y5=u(5);
    
end

y4=u(4);


y = [y1 y2 y3 y4 y5];

== matlab function detection_and_isolation_v3/MATLAB Function26 ==
  data: u input; y output; t input
function y = fcn(u,t)
y1=u(1);
y2=u(2);
if t>0.33
    y2=u(2)*1.32;
    y5=u(5)*1.52;
else
    y2=u(2);
    y5=u(5)*1.4;
      
end
y3=u(3);
y4=u(4);



y = [y1 y2 y3 y4 y5];

== matlab function detection_and_isolation_v3/MATLAB Function5 ==
  data: r input; rol output; x1 input; xp output; x input; m output
function [rol,xp,m]= fcn(r,x1,x)%u1,u2,ym1,ym2)
Th_det = 6.5e-8;
Th_det=0.1;  %2.5

tao1=0.0025;
tao2=0.0525;
m=x-x1;

% xp= r/tao1-x/tao1;

xp=0;

if m>0
    xp= r/tao1-x/tao1;
    Th_det=0.1;  %2.5
elseif m<0 && x<=0.8
    xp= r/tao2-x/tao2;
    Th_det=0.9; 
end



% sys=tf(1,[0.001 1]);


if x >=Th_det
    rol=1;
else
    rol=0;
end

== matlab function detection_and_isolation_v3/MATLAB Function6 ==
  data: r input; rol output; r1 input
function rol = fcn(r,r1)%u1,u2,ym1,ym2)
Th_det = 6.5e-8;
Th_det=0.1;  %2.5

m=r-r1;
if m>0
    Th_det=0.1;  %2.5
elseif m<0 && r<=0.1
    Th_det=0.9; 
end


% sys=tf(1,[0.001 1]);


if r >=Th_det
    rol=1;
else
    rol=0;
end

== matlab function detection_and_isolation_v3/MATLAB Function7 ==
  data: r input; rol output; r1 input; Th_det output
function [rol,Th_det] = fcn(r,r1)%u1,u2,ym1,ym2)
% Th_det = 6.5e-8;
Th_det=0.08;  %2.5

m=r-r1;
if m>0
    Th_det=0.07;%0.1;  %2.5
elseif m<0 && r<=0.007
    Th_det=0.9; 
end


% sys=tf(1,[0.001 1]);


if r >=Th_det
    rol=1;
else
    rol=0;
end

== matlab function detection_and_isolation_v3/MATLAB Function10 ==
  data: x_hat1 input; v1 output; x_hat2 input; x_hat3 input; x_hat4 input; ruo1 input; rol input
function v1 = fcn(x_hat1,x_hat2,x_hat3,x_hat4,ruo1,rol)

% yol=[u1 ; u2];
% ym=[ym1 ; ym2];
 C1=[0     1     0  0   0];
 v11=C1*(x_hat2'-x_hat1')*ruo1*rol;
 v12=C1*(x_hat2'-x_hat3')*ruo1*rol;
 v13=C1*(x_hat2'-x_hat4')*ruo1*rol;
 
 v1=(v11+v12+v13)/3;

== matlab function detection_and_isolation_v3/MATLAB Function11 ==
  data: x_hat1 input; v2 output; x_hat2 input; ruo2 input; rol input
function v2 = fcn(x_hat1,x_hat2,ruo2,rol)

% yol=[u1 ; u2];
% ym=[ym1 ; ym2];
 C2=[0     1     0];
 v2=C2*(x_hat2-x_hat1)*ruo2*rol;

== matlab function detection_and_isolation_v3/MATLAB Function8 ==
  data: ya input; ruo1 output; ym input
function ruo1 = fcn(ya,ym)
Th_uio_on = 3e-3;
Th_uio_off = 1e-5;


Th_uio_on = 6e-3;


% yol=[u1 ; u2];
% ym=[ym1 ; ym2];

% rd1=ya1-ym1;
% rd2=ya2-ym2;

% ya=[ya(1:3)y(5)];
r=ya-ym;

if abs(r(1))  >= Th_uio_on && abs(r(2))  <= Th_uio_off && abs(r(3))  <= Th_uio_off && abs(r(4))  <= Th_uio_off
    ruo1=1;
else
    ruo1=0;
end

== matlab function detection_and_isolation_v3/MATLAB Function9 ==
  data: ya input; ruo2 output; ym input
function ruo2 = fcn(ya,ym)
Th_uio_on = 3e-3;
Th_uio_off = 1e-5;


Th_uio_on = 6e-3;


% yol=[u1 ; u2];
% ym=[ym1 ; ym2];

% rd1=ya1-ym1;
% rd2=ya2-ym2;

% ya=[ya(1:3)y(5)];
r=ya-ym;

if abs(r(1))  >= Th_uio_on && abs(r(2))  <= Th_uio_off && abs(r(3))  <= Th_uio_off && abs(r(4))  <= Th_uio_off
    ruo2=1;
else
    ruo2=0;
end

== matlab function detection_and_isolation_v3/MATLAB Function12 ==
  data: ya input; ruo3 output; ym input
function ruo3 = fcn(ya,ym)
Th_uio_on = 3e-3;
Th_uio_off = 1e-5;


Th_uio_on = 6e-3;


% yol=[u1 ; u2];
% ym=[ym1 ; ym2];

% rd1=ya1-ym1;
% rd2=ya2-ym2;

% ya=[ya(1:3)y(5)];
r=ya-ym;

if abs(r(1))  >= Th_uio_on && abs(r(2))  <= Th_uio_off && abs(r(3))  <= Th_uio_off && abs(r(4))  <= Th_uio_off
    ruo3=1;
else
    ruo3=0;
end

== matlab function detection_and_isolation_v3/MATLAB Function13 ==
  data: ya input; ruo4 output; ym input
function ruo4 = fcn(ya,ym)
Th_uio_on = 3e-3;
Th_uio_off = 1e-5;


Th_uio_on = 6e-3;


% yol=[u1 ; u2];
% ym=[ym1 ; ym2];

% rd1=ya1-ym1;
% rd2=ya2-ym2;

% ya=[ya(1:3)y(5)];
r=ya-ym;

if abs(r(1))  >= Th_uio_on && abs(r(2))  <= Th_uio_off && abs(r(3))  <= Th_uio_off && abs(r(4))  <= Th_uio_off
    ruo4=1;
else
    ruo4=0;
end

== matlab function detection_and_isolation_v3/MATLAB Function27 ==
  data: u input; y output; t input
function y = fcn(u,t)
y1=u(1);
y2=u(2);
% if t>0.33
%     y2=u(2)*1.32;
%     y5=u(5)*1.52;
% else
%     y2=u(2);
%     y5=u(5)*1.4;
      
% end
y3=u(3);
y4=u(4);
y5=u(5);



y = [y1 y2 y3 y4 y5];

== matlab function detection_and_isolation_v3/MATLAB Function28 ==
  data: u input; y output; t input
function y = fcn(u,t)
y1=u(1);
y2=u(2);
if t>0.33
    y3=u(3)*0.54+5;
    y5=u(5)*1.14;
else
    y3=u(3)*0.7;
    y5=u(5);
      
end
% y3=u(3);
y4=u(4);



y = [y1 y2 y3 y4 y5];

== matlab function detection_and_isolation_v3/MATLAB Function29 ==
  data: u input; y output; t input
function y = fcn(u,t)
y1=u(1);
y2=u(2);
if t>0.33
    y3=u(3)*0.54;
%     y5=u(5)*1.14;
else
    y3=u(3)*0.7;
%     y5=u(5);
      
end
% y3=u(3);
y4=u(4);
y5=u(5);



y = [y1 y2 y3 y4 y5];

== matlab function detection_and_isolation_v3/MATLAB Function30 ==
  data: u input; y output; t input
function y = fcn(u,t)
y1=u(1);
y2=u(2);
% if t>0.33
%     y3=u(3)*0.54;
% %     y5=u(5)*1.14;
% else
%     y3=u(3)*0.7;
% %     y5=u(5);
%       
% end
y3=u(3);
y4=u(4);
y5=u(5);



y = [y1 y2 y3 y4 y5];

== matlab function detection_and_isolation_v3/MATLAB Function31 ==
  data: u input; y output; t input
function y = fcn(u,t)
y1=u(1);
y2=u(2);
if t>0.33
    y3=u(3)*0.54;
    y5=u(5)*1.13;
else
    y3=u(3)*0.7;
    y5=u(5);
      
end
% y3=u(3);
y4=u(4);
% y5=u(5);



y = [y1 y2 y3 y4 y5];

== matlab function detection_and_isolation_v3/MATLAB Function32 ==
  data: u input; y output; t input
function y = fcn(u,t)
y1=u(1); %-5  +5

if t>0.33
    y2=u(2)*1.27;
    
    y5=u(5)*1.47;
else
    y2=u(2);
    
    y5=u(5)*1.34;
    
end
y3=u(3);
y4=u(4);
% y5=u(5);



y = [y1 y2 y3 y4 y5];

== matlab function detection_and_isolation_v3/MATLAB Function33 ==
  data: u input; y output; t input
function y = fcn(u,t)
y1=u(1)-10;
y2=u(2);
if t>0.33
    y3=u(3)*0.54;
%     y5=u(5)*1.14;
else
    y3=u(3)*0.7;
%     y5=u(5);
      
end
% y3=u(3);
y4=u(4);
y5=u(5);



y = [y1 y2 y3 y4 y5];

== matlab function detection_and_isolation_v3/MATLAB Function34 ==
  settings: updateMethod=DISCRETE
  data: dr input; r output; t input
function r   = fcn(dr,t)
persistent a
if isempty(a)
    a=1;
       
end
if t<=0.33
    th=2.5e4;
%     v=2;
else
    th=4e4;
%     v=3;
end

r=0;
if a==2
    r=1;
end
% ra=r;

if abs(dr(2))>th
    r=1;
    a=a+1;
%     if v==0
%         v=1;
elseif abs(dr(2))>th && a==2
    r=0;
    a=1;
end


%     
% else
%     r=0;
% % elseif abs(dr(1))>=th
% %     r=0;
% %     v=0;
% end

== matlab function detection_and_isolation_v3/MATLAB Function35 ==
  settings: updateMethod=DISCRETE
  data: dr input; r output; t input
function r   = fcn(dr,t)
persistent a
if isempty(a)
    a=1;
       
end
if t<=0.33
    th=6.5e4;
%     v=2;
else
    th=8e4;
%     v=3;
end

r=0;
if a==2
    r=1;
end
% ra=r;

if abs(dr(3))>th
    r=1;
    a=a+1;
%     if v==0
%         v=1;
elseif abs(dr(3))>th && a==2
    r=0;
    a=1;
end


%     
% else
%     r=0;
% % elseif abs(dr(1))>=th
% %     r=0;
% %     v=0;
% end

== matlab function detection_and_isolation_v3/MATLAB Function36 ==
  data: dr input; r output; t input; ban input; c output; o output
function [r,c,o]   = fcn(dr,t,ban)

if t<=0.33
    th=2e4;
    %     v=2;
else
    th=4e4;
    %     v=3;
end

% r=0;
% c=1;

if ban==1
    r=1;
    c=0;
    if abs(dr(1))>th
        c=1;
        r=0;
    end
else
    r=0;
    c=1;
    if abs(dr(1))>th %%&& ban==0
        c=0;
        r=1;
    end
end

% ra=r;
% a=0;




% if abs(dr(1))>th && ban==1
%     %     a=10
%     c=1;
%     r=0;
%     % else
%     %     r=0;
%     %     c=1;
% end
% 
% if abs(dr(1))>th %%&& ban==0
%     %a=-1;
%     %     a=-10;
%     c=0;
%     r=1;
%     
% end





% if abs(dr(1))>th && ban==1
%     r=1;
%     c=0;
% %     if v==0
% %         v=1;
% elseif abs(dr(1))>th && ban==0
%     r=0;
%     c=1;
% else
%     r=0;
%     c=1;
% end
o=abs(dr(1));

== matlab function detection_and_isolation_v3/MATLAB Function37 ==
  settings: updateMethod=DISCRETE
  data: dr input; r output; t input; th output
function [r,th]   = fcn(dr,t)
persistent a
if isempty(a)
    a=1;
       
end
if t<=0.33
    th=2e4;
%     v=2;
else
    th=4e4;
%     v=3;
end

r=0;
if a==2
    r=1;
end
% ra=r;

if abs(dr(1))>th && a==1
    r=1;
    a=a+1;
%     if v==0
%         v=1;
elseif abs(dr(1))>th && a==2
    r=0;
    a=1;
end


%     
% else
%     r=0;
% % elseif abs(dr(1))>=th
% %     r=0;
% %     v=0;
% end

== matlab function detection_and_isolation_v3/MATLAB Function38 ==
  data: x_hat1 input; v1 output; x_hat2 input; x_hat3 input; x_hat4 input; ruo1 input; rol input
function v1 = fcn(x_hat1,x_hat2,x_hat3,x_hat4,ruo1,rol)

% yol=[u1 ; u2];
% ym=[ym1 ; ym2];
 C1=[1     0     0  0   0];
 v11=C1*(x_hat1'-x_hat2')*ruo1*rol;
 v12=C1*(x_hat1'-x_hat3')*ruo1*rol;
 v13=C1*(x_hat1'-x_hat4')*ruo1*rol;
 
 v1=(v11+v12+v13)/3;

== matlab function detection_and_isolation_v3/MATLAB Function39 ==
  data: x_hat1 input; v1 output; x_hat2 input; x_hat3 input; x_hat4 input; ruo1 input; rol input
function v1 = fcn(x_hat1,x_hat2,x_hat3,x_hat4,ruo1,rol)

% yol=[u1 ; u2];
% ym=[ym1 ; ym2];
 C1=[0     0     1  0   0];
 v11=C1*(x_hat3'-x_hat1')*ruo1*rol;
 v12=C1*(x_hat3'-x_hat2')*ruo1*rol;
 v13=C1*(x_hat3'-x_hat4')*ruo1*rol;
 
 v1=(v11+v12+v13)/3;
